simulink model "root"  (R2025b)
settings: Solver=VariableStepAuto  StartTime=0.0  StopTime=5  FixedStep=0.001  RelTol=1e-3
undefined symbols (not defined in the file or in its folder): deg, rad, s
libraries: eeGeneralControl x3, simulink_extras x2, aerolibconvert2 x1, slctrl_linear x1
settings Model: VariantFading=off  Creator=lew11  LastModifiedBy=rosette-nebula
settings ExplorerConfigSet: InternalSimMechanicsExplorerSettings=|
  | <ExplorerConfiguration>
  | 
  |   <canonicalview>default</canonicalview>
  | 
  |   <TilePanel>
  |     <TileInfo>
  |       <Tiles Columns="1" Count="1" Height="354" Rows="1" Width="500">
  |         <Row Weight="1"/>
  |         <Column Weight="1"/>
  |         <Tile Height="1" Width="1" X="0" Y="0"/>
  |       </Tiles>
  |     </TileInfo>
  |     <SceneInfo>
  |       <SceneViewer>
  |         <IsThisViewStd>
  |           <IsStandardView>off</IsStandardView>
  |           <StandardViewName>Front</StandardViewName>
  |         </IsThisViewStd>
  |         <BGColor>
  |           <R>1</R>
  |           <G>1</G>
  |           <B>1</B>
  |           <A>1</A>
  |         </BGColor>
  |         <Camera>
  |           <DoPerspective>on</DoPerspective>
  |           <Position>
  |             <X>0.42973179423875518</X>
  |             <Y>-1.6930026950929822</Y>
  |             <Z>0.046216126871379604</Z>
  |           </Position>
  |           <Center>
  |             <X>0</X>
  |             <Y>0</Y>
  |             <Z>-0.17316784451530964</Z>
  |           </Center>
  |           <Up>
  |             <X>-0.030659965459929769</X>
  |             <Y>0.1207902343997376</Y>
  |             <Z>0.99220445765560461</Z>
  |           </Up>
  |           <XLim>0.82089445238700331</XLim>
  |           <YLim>0.82089445238700331</YLim>
  |           <ViewLimDist>0.01</ViewLimDist>
  |         </Camera>
  |       </SceneViewer>
  |     </SceneInfo>
  |   </TilePanel>
  | 
  |   <MechEditorPanel>
  |     <GfxPanelCameraMap>
  |       <MapElement CameraMLId="Camera3" GfxPanelIndex="0"/>
  |     </GfxPanelCameraMap>
  |     <Cameras>
  |       <Camera>
  |         <Id>Camera1</Id>
  |         <Value>
  |           <Name>Body Cam</Name>
  |           <NativeCamera>
  |             <PositionTrackingFeature>Multibody_Sim.Body_Cam.R</PositionTrackingFeature>
  |             <CenterTrackingFeature>Multibody_Sim.COM_Ref.R</CenterTrackingFeature>
  |             <UpVectorTrackingFeature>Multibody_Sim.World.W</UpVectorTrackingFeature>
  |             <CenterTrackingOrigin>on</CenterTrackingOrigin>
  |             <UpVectorTrackingDirection>+Z</UpVectorTrackingDirection>
  |           </NativeCamera>
  |         </Value>
  |       </Camera>
  |       <Camera>
  |         <Id>Camera2</Id>
  |         <Value>
  |           <Name>Camera2</Name>
  |           <NativeCamera>
  |             <PositionKeyframeSet>
  |               <Keyframe>
  |                 <Time>0</Time>
  |                 <Value>
  |                   <X>0.11301</X>
  |                   <Y>-1.4589000000000001</Y>
  |                   <Z>0.22284999999999999</Z>
  |                 </Value>
  |               </Keyframe>
  |             </PositionKeyframeSet>
  |             <CenterKeyframeSet>
  |               <Keyframe>
  |                 <Time>0</Time>
  |                 <Value>
  |                   <X>0.11301</X>
  |                   <Y>-0.55457000000000001</Y>
  |                   <Z>0.22284999999999999</Z>
  |                 </Value>
  |               </Keyframe>
  |             </CenterKeyframeSet>
  |             <UpVectorKeyframeSet>
  |               <Keyframe>
  |                 <Time>0</Time>
  |                 <Value>
  |                   <X>0</X>
  |                   <Y>0</Y>
  |                   <Z>1</Z>
  |                 </Value>
  |               </Keyframe>
  |             </UpVectorKeyframeSet>
  |           </NativeCamera>
  |         </Value>
  |       </Camera>
  |       <Camera>
  |         <Id>Camera3</Id>
  |         <Value>
  |           <Name>ISO Downwards</Name>
  |           <NativeCamera>
  |             <PositionTrackingFeature>Multibody_Sim.TOP.Upper_Structure_Assembly_1_STEP_3_RIGID.F</PositionTrackingFeature>
  |             <CenterTrackingFeature>Multibody_Sim.Floor_R</CenterTrackingFeature>
  |             <UpVectorTrackingFeature>Multibody_Sim.Floor_R</UpVectorTrackingFeature>
  |             <CenterTrackingOrigin>on</CenterTrackingOrigin>
  |             <UpVectorTrackingDirection>+Z</UpVectorTrackingDirection>
  |           </NativeCamera>
  |         </Value>
  |       </Camera>
  |       <Camera>
  |         <Id>Camera4</Id>
  |         <Value>
  |           <Name>ISO tracking</Name>
  |           <NativeCamera>
  |             <PositionTrackingFeature>Multibody_Sim.World.W</PositionTrackingFeature>
  |             <CenterTrackingFeature>Multibody_Sim.COM_Ref_R</CenterTrackingFeature>
  |             <UpVectorTrackingFeature>Multibody_Sim.World_Frame.W</UpVectorTrackingFeature>
  |             <CenterTrackingOrigin>on</CenterTrackingOrigin>
  |             <UpVectorTrackingDirection>+Z</UpVectorTrackingDirection>
  |           </NativeCamera>
  |         </Value>
  |       </Camera>
  |     </Cameras>
  |     <VideoCreator>
  |       <IncludeTiles>All</IncludeTiles>
  |       <IncludeTime>on</IncludeTime>
  |       <IncludeWorldFrame>off</IncludeWorldFrame>
  |       <PlaybackSpeedRatio>1</PlaybackSpeedRatio>
  |       <FrameRate>30</FrameRate>
  |       <FrameSize>auto</FrameSize>
  |       <VideoFormat>UncompressedAVI</VideoFormat>
  |     </VideoCreator>
  |   </MechEditorPanel>
  | 
  |   <PlaybackSettings>
  |     <PlaybackSpeedFactor>1</PlaybackSpeedFactor>
  |   </PlaybackSettings>
  | 
  | </ExplorerConfiguration>

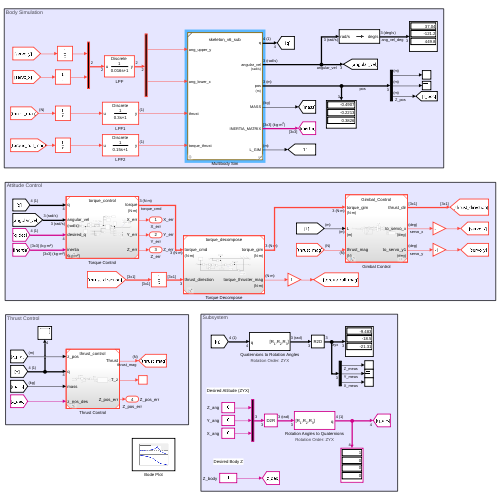
[thumbnail: Simulink's stored preview of the top-level diagram]
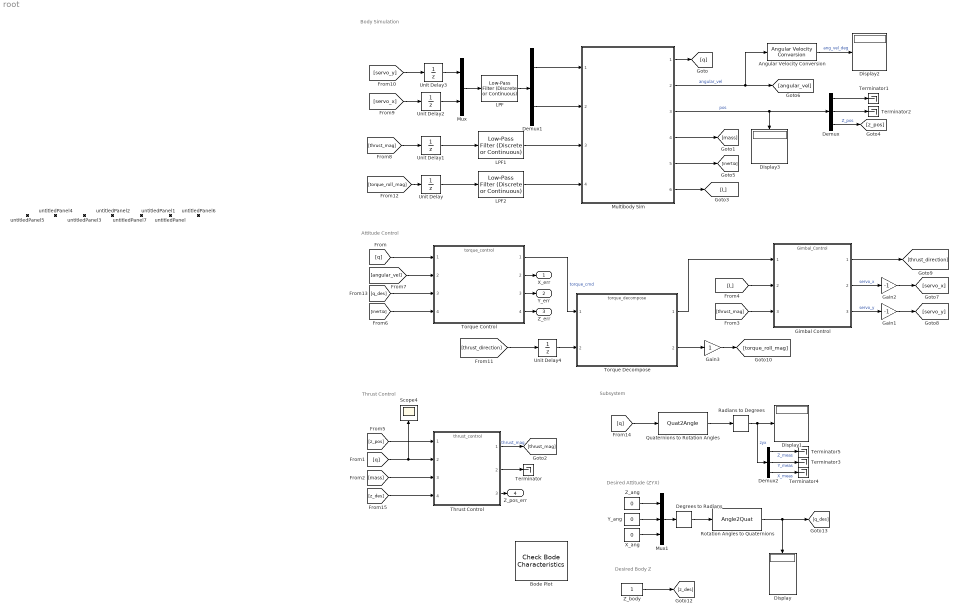
== system root ==
  note: Subsystem
  note: Body Simulation
  note: Attitude Control
  note: Thrust Control
  note: Desired Body Z
  note: Desired Attitude (ZYX)
  Angular Velocity Conversion : aerolibconvert2/Angular Velocity Conversion  IU=rad/s  OU=deg/s
  Bode Plot : slctrl_linear/Check Bode  Characteristics  InstantiateOnLoad=on  SaveOperatingPoints=off  LinearizationIOs={'/Z_ang', 1, 'in', 'off', '';'/Demux2', 1, 'out', 'off', ''}  LinearizeAt=SnapshotTimes  SnapshotTimes=[0 5 10 15 20 25]  TriggerType=rising  SampleTime=auto  RateConversionMethod=zoh  PreWarpFreq=10  UseExactDelayModel=off  UseFullBlockNameLabels=off  UseBusSignalLabels=off  enabled=on  stopWhenAssertionFail=off  export=off  ViewDlgPos=[100 237 510 390]  OpenViewOnLoad=off  LaunchViewOnOpen=off  FrequencyUnits=rad/s  MagnitudeUnits=dB  PhaseUnits=deg  TimeUnits=seconds  EnableUpperBound=off  UpperBoundFrequencies=[]  UpperBoundMagnitudes=[]  EnableLowerBound=off  LowerBoundFrequencies=[]  LowerBoundMagnitudes=[]
      settings: LibrarySourceBlock=slctrlblks/Linear Analysis Plots/Bode Plot  SaveToWorkspace=off  SaveName=sys
  Degrees to Radians : simulink_extras/Transformations/Degrees to Radians
  Demux : Demux  Outputs=3
  Demux1 : Demux  Outputs=2
  Demux2 : Demux  Outputs=3
  Display{,1..3} (4 alike) : Display
  Gain1 : Gain  Gain=-1
  Gain2 : Gain  Gain=-1
  Gain3 : Gain
  Gimbal Control : ModelReference  ModelNameDialog=Gimbal_Control.slx  SimulationMode=Normal  ModelReferenceVersion=1.55
  LPF : eeGeneralControl/Low-Pass Filter (Discrete or Continuous)  K=1  T=.016  B=inf  A=-inf  init_option=Inherited from block input  x0=0  Ts=-1
  LPF1 : eeGeneralControl/Low-Pass Filter (Discrete or Continuous)  K=1  T=.3  B=inf  A=-inf  init_option=Inherited from block input  x0=0  Ts=-1
  LPF2 : eeGeneralControl/Low-Pass Filter (Discrete or Continuous)  K=1  T=.15  B=inf  A=-inf  init_option=Inherited from block input  x0=0  Ts=-1
  Multibody Sim : Subsystem  ReferencedSubsystem=skeleton_v6_sub  initial_att=[0,0,0]  initial_ang_vel=[0,0,0]
  Mux : Mux  Inputs=2
  Mux1 : Mux  Inputs=3
  Quaternions to Rotation Angles : Quat2Angle
      settings: AttributesFormatString=Rotation Order: %<rotationOrder>
  Radians to Degrees : simulink_extras/Transformations/Radians to Degrees
  Rotation Angles to Quaternions : Angle2Quat
      settings: AttributesFormatString=Rotation Order: %<rotationOrder>
  Scope4 : Scope
      settings: ActiveDisplayYMinimum=-1.2826358132961515  ActiveDisplayYMaximum=1.391154513131281  DataLoggingVariableName=ScopeData11
  Terminator{,1..5} (6 alike) : Terminator
  Thrust Control : ModelReference  ModelNameDialog=thrust_control.slx  SimulationMode=Normal  ModelReferenceVersion=3.30
  Torque Control : ModelReference  ModelNameDialog=torque_control.slx  SimulationMode=Normal  ModelReferenceVersion=1.119
  Torque Decompose : ModelReference  ModelNameDialog=torque_decompose.slx  SimulationMode=Normal  ModelReferenceVersion=1.40
  Unit Delay{,1..3} (4 alike) : UnitDelay  SampleTime=-1  HasFrameUpgradeWarning=on
  Unit Delay4 : UnitDelay  InitialCondition=[0; 0; -1]  SampleTime=-1  HasFrameUpgradeWarning=on
  X_ang : Constant  Value=0
  Y_ang : Constant  Value=0
  Z_ang : Constant  Value=0
  Z_body : Constant
  untitledPanel : Subsystem  Tag=HiddenForWebPanel  IsWebBlockPanel=on
  untitledPanel1 : Subsystem  Tag=HiddenForWebPanel  IsWebBlockPanel=on
  untitledPanel2 : Subsystem  Tag=HiddenForWebPanel  IsWebBlockPanel=on
  untitledPanel3 : Subsystem  Tag=HiddenForWebPanel  IsWebBlockPanel=on
  untitledPanel4 : Subsystem  Tag=HiddenForWebPanel  IsWebBlockPanel=on
  untitledPanel5 : Subsystem  Tag=HiddenForWebPanel  IsWebBlockPanel=on
  untitledPanel6 : Subsystem  Tag=HiddenForWebPanel  IsWebBlockPanel=on
  untitledPanel7 : Subsystem  Tag=HiddenForWebPanel  IsWebBlockPanel=on
  X_err : Outport  SignalName=X_err
  Y_err : Outport  Port=2  SignalName=Y_err
  Z_err : Outport  Port=3  SignalName=Z_err
  Z_pos_err : Outport  Port=4  SignalName=Z_pos_err
  wires:
  Thrust Control/2 -> Terminator/1
  [z_pos] -> Thrust Control/1
  Thrust Control/1 -> [thrust_mag]  "thrust_mag"
  [mass] -> Thrust Control/3
  [q] -> Thrust Control/2, Scope4/1
  [z_des] -> Thrust Control/4
  [q] -> Torque Control/1
  Gimbal Control/3 -> Gain1/1  "servo_y"
  Torque Control/1 -> Torque Decompose/1  "torque_cmd"
  [angular_vel] -> Torque Control/2
  Torque Decompose/1 -> Gimbal Control/1
  Torque Decompose/2 -> Gain3/1
  Gain2/1 -> [servo_x]
  [thrust_direction] -> Unit Delay4/1
  Unit Delay4/1 -> Torque Decompose/2
  [thrust_mag] -> Gimbal Control/3
  Gain3/1 -> [torque_roll_mag]
  Gain1/1 -> [servo_y]
  Gimbal Control/1 -> [thrust_direction]
  [L] -> Gimbal Control/2
  Gimbal Control/2 -> Gain2/1  "servo_x"
  [inertia] -> Torque Control/4
  [q_des] -> Torque Control/3
  Unit Delay1/1 -> LPF1/1
  Demux/3 -> [z_pos]  "Z_pos"
  Multibody Sim/2 -> Angular Velocity Conversion/1, [angular_vel]  "angular_vel"
  [servo_x] -> Unit Delay2/1
  LPF1/1 -> Multibody Sim/3
  [torque_roll_mag] -> Unit Delay/1
  Multibody Sim/1 -> [q]
  Unit Delay2/1 -> Mux/2
  Multibody Sim/6 -> [L]
  Multibody Sim/3 -> Display3/1, Demux/1  "pos"
  Angular Velocity Conversion/1 -> Display2/1  "ang_vel_deg"
  Multibody Sim/5 -> [inertia]
  Unit Delay3/1 -> Mux/1
  [thrust_mag] -> Unit Delay1/1
  LPF2/1 -> Multibody Sim/4
  Unit Delay/1 -> LPF2/1
  Demux1/1 -> Multibody Sim/1
  Multibody Sim/4 -> [mass]
  Demux1/2 -> Multibody Sim/2
  Mux/1 -> LPF/1
  Demux/2 -> Terminator2/1
  [servo_y] -> Unit Delay3/1
  Demux/1 -> Terminator1/1
  LPF/1 -> Demux1/1
  X_ang/1 -> Mux1/3
  Mux1/1 -> Degrees to Radians/1
  Z_body/1 -> [z_des]
  Demux2/1 -> Terminator5/1  "Z_meas"
  Quaternions to Rotation Angles/1 -> Radians to Degrees/1
  Degrees to Radians/1 -> Rotation Angles to Quaternions/1
  Z_ang/1 -> Mux1/1
  Radians to Degrees/1 -> Demux2/1, Display1/1  "zyx"
  Rotation Angles to Quaternions/1 -> [q_des], Display/1
  [q] -> Quaternions to Rotation Angles/1
  Y_ang/1 -> Mux1/2
  Demux2/2 -> Terminator3/1  "Y_meas"
  Demux2/3 -> Terminator4/1  "X_meas"
  Thrust Control/3 -> Z_pos_err/1
  Torque Control/2 -> X_err/1
  Torque Control/3 -> Y_err/1
  Torque Control/4 -> Z_err/1

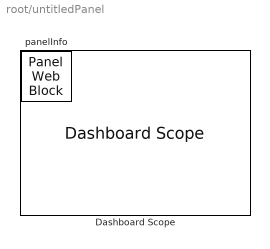
== system root/untitledPanel ==
  Dashboard Scope : DashboardScope  Tag=HiddenForWebPanel  PanelInfo="{\"height\":239,\"left\":14,\"panelId\":\"panelId-df574acb-9b53-4ca6-ae86-6ba3631c2ba2\",\"top\":14,\"type\":\"panelChild\",\"version\":\"2019b\",\"width\":376,\"zIndex\":1500002}"  FontColor=[0.0, 0.0, 0.0]
  panelInfo : PanelWebBlock  Tag=HiddenForWebPanel  PanelInfo="{\"compacted\":true,\"height\":270,\"isActiveTab\":false,\"left\":17,\"name\":\"Thrust Mag\",\"panelId\":\"panelId-df574acb-9b53-4ca6-ae86-6ba3631c2ba2\",\"tabIndex\":3,\"tabbedSetId\":\"tabbedSet0758760287\",\"top\":449,\"type\":\"panel\",\"version\":\"2019b\",\"visible\":false,\"width\":411,\"zIndex\":1500008}"  PanelSnapshot=<binary blob, 10360 chars, not shown>

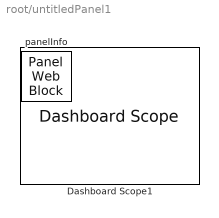
== system root/untitledPanel1 ==
  Dashboard Scope1 : DashboardScope  Tag=HiddenForWebPanel  PanelInfo="{\"height\":238,\"left\":14,\"panelId\":\"panelId-f5ddd5ba-68bf-4bce-b4ed-3ca48cb51992\",\"top\":11,\"type\":\"panelChild\",\"version\":\"2019b\",\"width\":384,\"zIndex\":1500002}"  FontColor=[0.0, 0.0, 0.0]
  panelInfo : PanelWebBlock  Tag=HiddenForWebPanel  PanelInfo="{\"compacted\":true,\"height\":270,\"isActiveTab\":false,\"left\":17,\"name\":\"Angular Vel\",\"panelId\":\"panelId-f5ddd5ba-68bf-4bce-b4ed-3ca48cb51992\",\"tabIndex\":4,\"tabbedSetId\":\"tabbedSet0758760287\",\"top\":449,\"type\":\"panel\",\"version\":\"2019b\",\"visible\":false,\"width\":411,\"zIndex\":1500018}"  PanelSnapshot=<binary blob, 37536 chars, not shown>

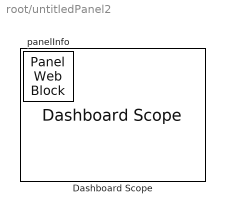
== system root/untitledPanel2 ==
  Dashboard Scope : DashboardScope  Tag=HiddenForWebPanel  PanelInfo="{\"height\":287,\"left\":15,\"panelId\":\"panelId-bf281c9f-ba11-4427-b965-b4cc8690ae3f\",\"top\":15,\"type\":\"panelChild\",\"version\":\"2019b\",\"width\":503,\"zIndex\":1500002}"  LegendPosition=InsideTop  FontColor=[0.0, 0.0, 0.0]
  panelInfo : PanelWebBlock  Tag=HiddenForWebPanel  PanelInfo="{\"compacted\":true,\"height\":319,\"isActiveTab\":true,\"left\":17,\"name\":\"Pos\",\"panelId\":\"panelId-bf281c9f-ba11-4427-b965-b4cc8690ae3f\",\"tabIndex\":0,\"tabbedSetId\":\"tabbedSet0758760287\",\"top\":449,\"type\":\"panel\",\"version\":\"2019b\",\"visible\":true,\"width\":545,\"zIndex\":1500006}"  PanelSnapshot=<binary blob, 42560 chars, not shown>

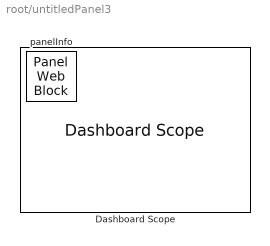
== system root/untitledPanel3 ==
  Dashboard Scope : DashboardScope  Tag=HiddenForWebPanel  PanelInfo="{\"height\":244,\"left\":9,\"panelId\":\"panelId-bc59ce79-e06d-46e6-8976-fc32dab224ce\",\"top\":11,\"type\":\"panelChild\",\"version\":\"2019b\",\"width\":384,\"zIndex\":1500002}"  LegendPosition=InsideTop  FontColor=[0.0, 0.0, 0.0]
  panelInfo : PanelWebBlock  Tag=HiddenForWebPanel  PanelInfo="{\"compacted\":true,\"height\":270,\"isActiveTab\":false,\"left\":17,\"name\":\"Torque Cmd\",\"panelId\":\"panelId-bc59ce79-e06d-46e6-8976-fc32dab224ce\",\"tabIndex\":2,\"tabbedSetId\":\"tabbedSet0758760287\",\"top\":449,\"type\":\"panel\",\"version\":\"2019b\",\"visible\":false,\"width\":411,\"zIndex\":1500010}"  PanelSnapshot=<binary blob, 15968 chars, not shown>

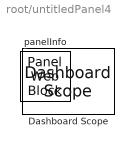
== system root/untitledPanel4 ==
  Dashboard Scope : DashboardScope  Tag=HiddenForWebPanel  PanelInfo="{\"height\":302,\"left\":19,\"panelId\":\"panelId-afeff753-055c-4466-a3b4-b1d4746a0976\",\"top\":21,\"type\":\"panelChild\",\"version\":\"2019b\",\"width\":485,\"zIndex\":1500002}"  FontColor=[0.0, 0.0, 0.0]
  panelInfo : PanelWebBlock  Tag=HiddenForWebPanel  PanelInfo="{\"compacted\":true,\"height\":348,\"isActiveTab\":false,\"left\":17,\"name\":\"Gimbal\",\"panelId\":\"panelId-afeff753-055c-4466-a3b4-b1d4746a0976\",\"tabIndex\":5,\"tabbedSetId\":\"tabbedSet0758760287\",\"top\":449,\"type\":\"panel\",\"version\":\"2019b\",\"visible\":false,\"width\":530,\"zIndex\":1500014}"  PanelSnapshot=<binary blob, 16760 chars, not shown>

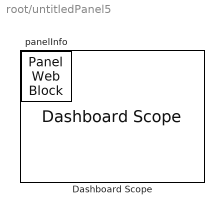
== system root/untitledPanel5 ==
  Dashboard Scope : DashboardScope  Tag=HiddenForWebPanel  PanelInfo="{\"height\":305,\"left\":18,\"panelId\":\"panelId-73bbacd2-b43c-49af-8a25-33fa81718205\",\"top\":18,\"type\":\"panelChild\",\"version\":\"2019b\",\"width\":549,\"zIndex\":1500002}"  FontColor=[0.0, 0.0, 0.0]
  panelInfo : PanelWebBlock  Tag=HiddenForWebPanel  PanelInfo="{\"compacted\":true,\"height\":346,\"isActiveTab\":false,\"left\":17,\"name\":\"Attitude\",\"panelId\":\"panelId-73bbacd2-b43c-49af-8a25-33fa81718205\",\"tabIndex\":1,\"tabbedSetId\":\"tabbedSet0758760287\",\"top\":449,\"type\":\"panel\",\"version\":\"2019b\",\"visible\":false,\"width\":589,\"zIndex\":1500016}"  PanelSnapshot=<binary blob, 65508 chars, not shown>

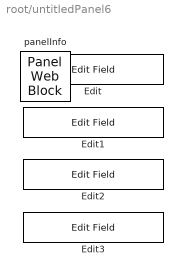
== system root/untitledPanel6 ==
  Edit : EditField  Tag=HiddenForWebPanel  PanelInfo="{\"height\":39,\"left\":174,\"panelId\":\"panelId-3babcc67-e047-4488-9d66-89986165da81\",\"top\":41,\"type\":\"panelChild\",\"version\":\"2019b\",\"width\":186,\"zIndex\":1500004}"  LabelPosition=Hide  ShowInitialText=on  Alignment=Center
  Edit1 : EditField  Tag=HiddenForWebPanel  PanelInfo="{\"height\":39,\"left\":174,\"panelId\":\"panelId-3babcc67-e047-4488-9d66-89986165da81\",\"top\":97,\"type\":\"panelChild\",\"version\":\"2019b\",\"width\":186,\"zIndex\":1500008}"  LabelPosition=Hide  ShowInitialText=on  Alignment=Center
  Edit2 : EditField  Tag=HiddenForWebPanel  PanelInfo="{\"height\":39,\"left\":175,\"panelId\":\"panelId-3babcc67-e047-4488-9d66-89986165da81\",\"top\":161,\"type\":\"panelChild\",\"version\":\"2019b\",\"width\":186,\"zIndex\":1500006}"  LabelPosition=Hide  ShowInitialText=on  Alignment=Center
  Edit3 : EditField  Tag=HiddenForWebPanel  PanelInfo="{\"height\":39,\"left\":175,\"panelId\":\"panelId-3babcc67-e047-4488-9d66-89986165da81\",\"top\":223,\"type\":\"panelChild\",\"version\":\"2019b\",\"width\":186,\"zIndex\":1500002}"  LabelPosition=Hide  ShowInitialText=on  Alignment=Center
  panelInfo : PanelWebBlock  Tag=HiddenForWebPanel  PanelInfo="{\"compacted\":true,\"height\":343,\"isActiveTab\":true,\"labels\":{\"label0760470857\":{\"deleted\":false,\"left\":27,\"settings\":{\"backgroundColor\":\"rgba(0, 0, 0, 0)\",\"bold\":false,\"font\":\"Arial\",\"fontColor\":\"black\",\"fontSize\":1.19,\"italicized\":false,\"underlined\":false},\"text\":\"Z-axis Angle\",\"top\":50},\"label1202873996\":{\"deleted\":false,\"left\":30,\"settings\":{\"backgroundColor\":\"rgba(0, 0, 0, 0)\",\"bold\":false,\"font\":\"Arial\",\"fontColor\":\"black\",\"fontSize\":1.19,\"italicized\":false,\"underlined\":false},\"text\":\"Y-Axis Angle\",\"top\":106},\"label6086478585\":{\"deleted\":false,\"left\":31,\"settings\":{\"backgroundColor\":\"rgba(0, 0, 0, 0)\",\"bold\":false,\"font\":\"Arial\",\"fontColor\":\"black\",\"fontSize\":1.19,\"italicized\":false,\"underlined\":false},\"text\":\"Desired Height\",\"top\":236},\"label8074754192\":{\"deleted\":false,\"left\":31,\"settings\":{\"backgroundColor\":\"rgba(0, 0, 0, 0)\",\"bold\":false,\"font\":\"Arial\",\"fontColor\":\"black\",\"fontSize\":1.19,\"italicized\":false,\"underlined\":false},\"text\":\"X-Axis Angle\",\"top\":167}},\"left\":14,\"name\":\"Desired Parameters\",\"panelId\":\"panelId-3babcc67-e047-4488-9d66-89986165da81\",\"tabIndex\":0,\"tabbedSetId\":\"tabbedSet5976375065\",\"top\":109,\"type\":\"panel\",\"version\":\"2019b\",\"visible\":true,\"width\":388,\"zIndex\":1500020}"  PanelSnapshot=<binary blob, 20484 chars, not shown>

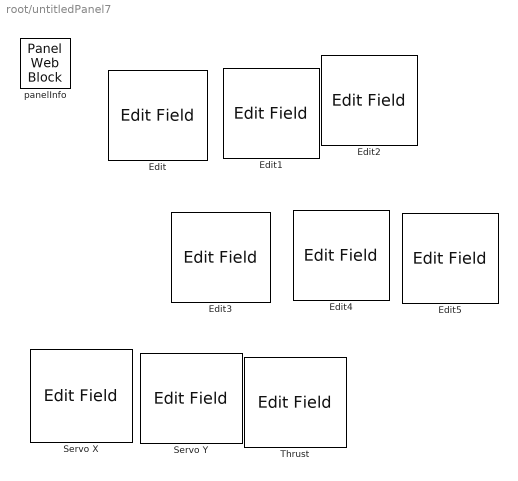
== system root/untitledPanel7 ==
  Edit : EditField  Tag=HiddenForWebPanel  PanelInfo="{\"height\":68,\"left\":21,\"panelId\":\"panelId-9a0878ef-bd6a-447e-860e-43c9df46bd55\",\"top\":39,\"type\":\"panelChild\",\"version\":\"2019b\",\"width\":75,\"zIndex\":1500002}"  LabelPosition=Hide  ShowInitialText=on  Alignment=Center
  Edit1 : EditField  Tag=HiddenForWebPanel  PanelInfo="{\"height\":68,\"left\":100,\"panelId\":\"panelId-9a0878ef-bd6a-447e-860e-43c9df46bd55\",\"top\":38,\"type\":\"panelChild\",\"version\":\"2019b\",\"width\":73,\"zIndex\":1500004}"  LabelPosition=Hide  ShowInitialText=on  Alignment=Center
  Edit2 : EditField  Tag=HiddenForWebPanel  PanelInfo="{\"height\":68,\"left\":180,\"panelId\":\"panelId-9a0878ef-bd6a-447e-860e-43c9df46bd55\",\"top\":38,\"type\":\"panelChild\",\"version\":\"2019b\",\"width\":73,\"zIndex\":1500006}"  LabelPosition=Hide  ShowInitialText=on  Alignment=Center
  Edit3 : EditField  Tag=HiddenForWebPanel  PanelInfo="{\"height\":68,\"left\":23,\"panelId\":\"panelId-9a0878ef-bd6a-447e-860e-43c9df46bd55\",\"top\":151,\"type\":\"panelChild\",\"version\":\"2019b\",\"width\":75,\"zIndex\":1500008}"  LabelPosition=Hide  ShowInitialText=on  Alignment=Center
  Edit4 : EditField  Tag=HiddenForWebPanel  PanelInfo="{\"height\":68,\"left\":104,\"panelId\":\"panelId-9a0878ef-bd6a-447e-860e-43c9df46bd55\",\"top\":151,\"type\":\"panelChild\",\"version\":\"2019b\",\"width\":73,\"zIndex\":1500010}"  LabelPosition=Hide  ShowInitialText=on  Alignment=Center
  Edit5 : EditField  Tag=HiddenForWebPanel  PanelInfo="{\"height\":68,\"left\":183,\"panelId\":\"panelId-9a0878ef-bd6a-447e-860e-43c9df46bd55\",\"top\":151,\"type\":\"panelChild\",\"version\":\"2019b\",\"width\":73,\"zIndex\":1500012}"  LabelPosition=Hide  ShowInitialText=on  Alignment=Center
  Servo X : EditField  Tag=HiddenForWebPanel  PanelInfo="{\"height\":70,\"left\":20,\"panelId\":\"panelId-9a0878ef-bd6a-447e-860e-43c9df46bd55\",\"top\":260,\"type\":\"panelChild\",\"version\":\"2019b\",\"width\":76,\"zIndex\":1500016}"  LabelPosition=Hide  ShowInitialText=on  Alignment=Center
  Servo Y : EditField  Tag=HiddenForWebPanel  PanelInfo="{\"height\":70,\"left\":105,\"panelId\":\"panelId-9a0878ef-bd6a-447e-860e-43c9df46bd55\",\"top\":261,\"type\":\"panelChild\",\"version\":\"2019b\",\"width\":76,\"zIndex\":1500018}"  LabelPosition=Hide  ShowInitialText=on  Alignment=Center
  Thrust : EditField  Tag=HiddenForWebPanel  PanelInfo="{\"height\":69,\"left\":187,\"panelId\":\"panelId-9a0878ef-bd6a-447e-860e-43c9df46bd55\",\"top\":262,\"type\":\"panelChild\",\"version\":\"2019b\",\"width\":70,\"zIndex\":1500014}"  LabelPosition=Hide  ShowInitialText=on  Alignment=Center
  panelInfo : PanelWebBlock  Tag=HiddenForWebPanel  PanelInfo="{\"compacted\":true,\"height\":352,\"isActiveTab\":false,\"labels\":{\"label2638262863\":{\"deleted\":false,\"left\":17,\"settings\":{\"backgroundColor\":\"rgba(0, 0, 0, 0)\",\"bold\":false,\"font\":\"Arial\",\"fontColor\":\"black\",\"fontSize\":0.97,\"italicized\":false,\"underlined\":false},\"text\":\"Initial Angular Velocity (X, Y, Z)\",\"top\":125},\"label3097643195\":{\"deleted\":false,\"left\":38,\"settings\":{\"backgroundColor\":\"rgba(0, 0, 0, 0)\",\"bold\":false,\"font\":\"Arial\",\"fontColor\":\"black\",\"fontSize\":0.68,\"italicized\":false,\"underlined\":false},\"text\":\"Servo X\",\"top\":247},\"label5225599841\":{\"deleted\":false,\"left\":18,\"settings\":{\"backgroundColor\":\"rgba(0, 0, 0, 0)\",\"bold\":false,\"font\":\"Arial\",\"fontColor\":\"black\",\"fontSize\":0.97,\"italicized\":false,\"underlined\":false},\"text\":\"Initial Attitude (X, Y, Z)\",\"top\":14},\"label7229011160\":{\"deleted\":false,\"left\":182,\"settings\":{\"backgroundColor\":\"rgba(0, 0, 0, 0)\",\"bold\":false,\"font\":\"Arial\",\"fontColor\":\"black\",\"fontSize\":0.68,\"italicized\":false,\"underlined\":false},\"text\":\"Thrust Magnitude\",\"top\":247},\"label8889389468\":{\"deleted\":false,\"left\":119,\"settings\":{\"backgroundColor\":\"rgba(0, 0, 0, 0)\",\"bold\":false,\"font\":\"Arial\",\"fontColor\":\"black\",\"fontSize\":0.68,\"italicized\":false,\"underlined\":false},\"text\":\"Servo Y\",\"top\":247}},\"left\":14,\"name\":\"Initial Conditions\",\"panelId\":\"panelId-9a0878ef-bd6a-447e-860e-43c9df46bd55\",\"tabIndex\":1,\"tabbedSetId\":\"tabbedSet5976375065\",\"top\":109,\"type\":\"panel\",\"version\":\"2019b\",\"visible\":false,\"width\":300,\"zIndex\":1500022}"  PanelSnapshot=<binary blob, 17760 chars, not shown>
